simulink model "Mmc"  (R2024b)
settings: Solver=ode23t  StartTime=0.0  StopTime=2  FixedStep=Ts_Power
values from neighbouring files (symbols this model uses):
  Ch = 0.94e-6*ones(4,3)    [MmcParameters.m]
  Cm = 0.55e-3    (= 0.00055)    [MmcParameters.m]
  Cmo = 0.55e-3*ones(4,3)    [MmcParameters.m]
  eta = N*delta_wmax*Vmax^2/(P_rated*sin(phi_r)-Q_rated*cos(phi_r))    [MmcParameters.m]
  Fnom = 50    [MmcParameters.m]
  fs = 20000    [MmcParameters.m]
  I_b = Snom/Vnom_AC/sqrt(3)    [MmcParameters.m]
  Ipp_b = Snom/Vnom_AC/sqrt(3/2)    [MmcParameters.m]
  kicir = R0*alpha_ic    (= 62831.8530718)    [MmcParameters.m]
  kpcir = L0*alpha_ic    (= 1012.64003201)    [MmcParameters.m]
  L0 = (4.67e-3+5e-3)    (= 0.00967)    [MmcParameters.m]
  mu = eta*4/((2*Vmax^2-V0^2)^2-V0^4)*(P_rated*cos(phi_r)+Q_rated*sin(phi_r))/N    [MmcParameters.m]
  Nb_PM = 2    [MmcParameters.m]
  phi_r = pi/2    (= 1.57079632679)    [MmcParameters.m]
  R0 = 0.1+0.5    (= 0.6)    [MmcParameters.m]
  Rdis = 1e6*ones(4,3)    [MmcParameters.m]
  Rh = 1e-3./(2*pi*1000*Ch)    [MmcParameters.m]
  Rm = 0.2./(2*pi*120*Cmo)    [MmcParameters.m]
  SCR = 10    [MmcParameters.m]
  SigmaM = 10    [MmcParameters.m]
  Snom = 20*Vnom_AC*sqrt(3)    [MmcParameters.m]
  Ts_Power = 5e-7    (= 5e-07)    [MmcParameters.m]
  V0 = 1    [MmcParameters.m]
  V_b = Vnom_AC    (= 400)    [MmcParameters.m]
  VDCm = 480/2    (= 240)    [MmcParameters.m]
  VDCp = 480/2    (= 240)    [MmcParameters.m]
  Vnom_AC = 400    [MmcParameters.m]
  Vnom_PM = 480/2    (= 240)    [MmcParameters.m]
  w_b = 2*pi*Fnom    (= 314.159265359)    [MmcParameters.m]
  Zn = Vnom_AC^2 / Snom    [MmcParameters.m]
undefined symbols (not defined in the file or in its folder): DiscIntNeverNeededParam
libraries: spsIGBTDiodeLib x48, spsSeriesRLCBranchLib x42, spsVoltageMeasurementLib x16, spsTriangleGeneratorLib x12, spsCurrentMeasurementLib x7, spsFirstOrderFilterLib x6, eePwmGeneratorMultilevel x6, spsabctodq0Lib x3, spsGroundLib x2, spsMeanLib x2, spsDCVoltageSourceLib x2, spsThreePhaseVIMeasurementLib x2
(part 1 of 3)
settings Model: Creator=The MathWorks, Inc.  LastModifiedBy=isabe
settings SolverCC: AlgebraicLoopSolver=TrustRegion
settings DataIOCC: SaveFormat=StructureWithTime  SaveOutput=off  SignalLogging=off  DSMLogging=off  SaveTime=off  ReturnWorkspaceOutputs=off
settings OptimizationCC: ExpressionDepthLimit=2147483647  LifeSpan=inf
settings DebuggingCC: UnderspecifiedInitializationDetection=Classic  MergeDetectMultiDrivingBlocksExec=none  SolverPrmCheckMsg=warning  FcnCallInpInsideContextMsg=warning  UnconnectedInputMsg=warning  UnconnectedOutputMsg=warning  UnconnectedLineMsg=warning  AllowSymbolicDim=off  StateNameClashWarn=warning  SFUnexpectedBacktrackingDiag=warning  SFNoUnconditionalDefaultTransitionDiag=warning  SFExecutionAtInitializationDiag=none  ArithmeticOperatorsInVariantConditions=warning
settings HardwareCC: ProdBitPerPointer=32  ProdBitPerSizeT=32  ProdBitPerPtrDiffT=32  ProdLargestAtomicFloat=None  ProdIntDivRoundTo=Undefined  ProdEndianess=Unspecified  ProdWordSize=32  ProdHWDeviceType=32-bit Generic
settings ModelReferenceCC: EnableRefExpFcnMdlSchedulingChecks=on  PropagateSignalLabelsOutOfModel=off
settings SFSimCC: SimUseLocalCustomCode=off  CustomCodeUndefinedFunction=UseInterfaceOnly
settings RTWCC: RTWUseLocalCustomCode=off  GPUComputeCapability=3.5
settings CodeAppCC: StateflowObjectComments=on
settings GRTTargetCC: TargetLangStandard=C89/C90 (ANSI)  CombineOutputUpdateFcns=off  GRTInterface=on
settings ConfigComp: CovMetricSettings=dw  CovSaveCumulativeToWorkspaceVar=on  CovSaveSingleToWorkspaceVar=on  CovExternalEMLEnable=off
settings SimscapeCC: SimscapeNormalizeSystem=off  SimscapeNominalValues={1, 'bar'; 1, 'cm^3/s'; 1, 'bar*kg/s'; 1, 'kJ/kg'; 1, 'kW'; }

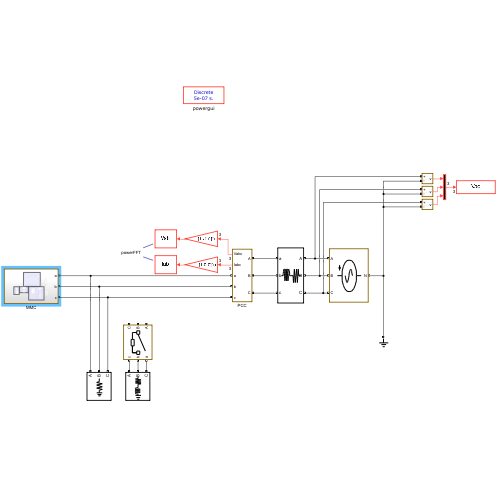
[thumbnail: Simulink's stored preview of the top-level diagram]
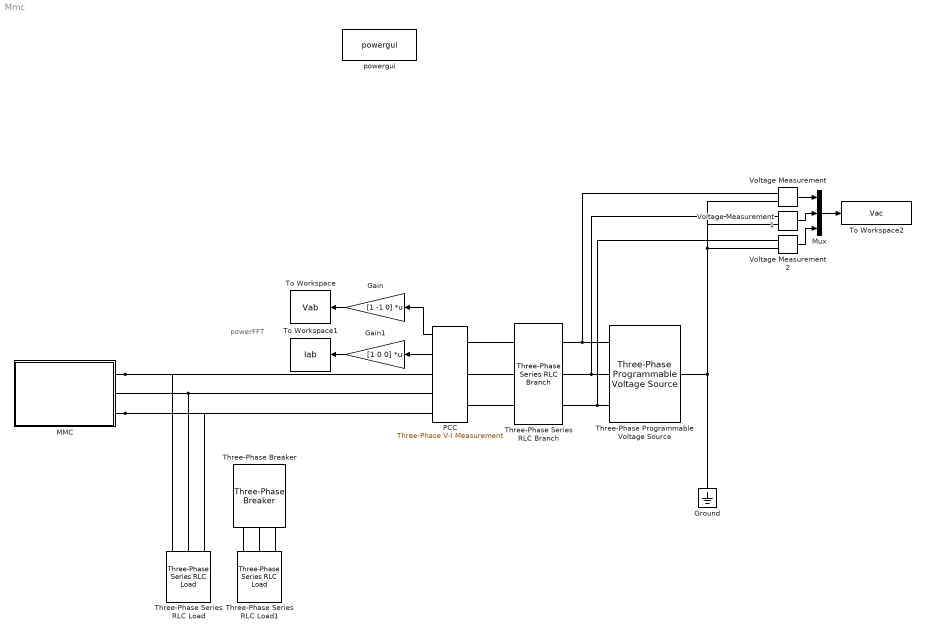
== system Mmc ==
  note: powerFFT
  Gain : Gain  Gain=[1 -1 0]  Multiplication=Matrix(K*u)
  Gain1 : Gain  Gain=[1 0 0]  Multiplication=Matrix(K*u)
  Ground : spsGroundLib/Ground  LConnTagsString=a
  MMC : Subsystem
  Mux : Mux  Inputs=3
  PCC : spsThreePhaseVIMeasurementLib/Three-Phase V-I Measurement  VoltageMeasurement=phase-to-ground  SetLabelV=off  LabelV=Vabc  Vpu=on  VpuLL=off  CurrentMeasurement=yes  SetLabelI=off  LabelI=Iabc  Ipu=on  Pbase=Snom  Vbase=Vnom_AC  OutputType=Complex  PhasorSimulation=off  PSBequivalent=0
  Three-Phase Programmable Voltage Source : spsThreePhaseProgrammableVoltageSourceLib/Three-Phase Programmable Voltage Source  PositiveSequence="[Vnom_AC  0 Fnom]"  VariationEntity=None  VariationType=Step  VariationTypeAlt=Step  VariationStep=-0.7  VariationRate=5  VariationMagnitude=0.3  VariationFrequency=2  VariationTiming=[1 17]  VariationPhaseA=off  Amplitudes=[1 0.8 1.2 1.0]  TimeValues=[0 0.1 0.15 0.2]  HarmonicGeneration=off  HarmonicA=[3 0.2 -25 0]  HarmonicB=[2 0.15 35 2]  Timing="[0.05  3]"  BusType=swing  Pref=0  Qref=0  Qmin=-inf  Qmax=inf
  Three-Phase Series RLC Branch : spsThreePhaseSeriesRLCBranchLib/Three-Phase Series RLC Branch  LConnTagsString=A|B|C  RConnTagsString=A|B|C  BranchType=RL  Resistance=Zn/SCR/sqrt(101)  Inductance=Zn/SCR/2/pi/Fnom*10/sqrt(101)  Capacitance=1e-6  Measurements=None
  Three-Phase Series RLC Load : spsThreePhaseSeriesRLCLoadLib/Three-Phase Series RLC Load  LConnTagsString=A|B|C  Configuration=Y (grounded)  NominalVoltage=Vnom_AC  Vabc=[1e3 1e3 1e3]  Vabcp=[1e3 1e3 1e3]  NominalFrequency=Fnom  UnbalancedPower=off  ActivePower=Snom*.05  InductivePower=Snom*.0  CapacitivePower=0  Pabc=[10e3 9e3 11e3]  QLabc=[100 90 110]  QCabc=[100 90 110]  Pabcp=[10e3 9e3 11e3]  QLabcp=[100 90 110]  QCabcp=[100 90 110]  Measurements=None  LoadType=constant Z
  Three-Phase Series RLC Load1 : spsThreePhaseSeriesRLCLoadLib/Three-Phase Series RLC Load  LConnTagsString=A|B|C  Configuration=Y (grounded)  NominalVoltage=Vnom_AC  Vabc=[1e3 1e3 1e3]  Vabcp=[1e3 1e3 1e3]  NominalFrequency=Fnom  UnbalancedPower=off  ActivePower=Snom*.25  InductivePower=Snom*.2  CapacitivePower=0  Pabc=[10e3 9e3 11e3]  QLabc=[100 90 110]  QCabc=[100 90 110]  Pabcp=[10e3 9e3 11e3]  QLabcp=[100 90 110]  QCabcp=[100 90 110]  Measurements=None  LoadType=constant PQ
  Three-Phase Breaker : spsThreePhaseBreakerLib/Three-Phase Breaker  InitialState=open  SwitchA=on  SwitchB=on  SwitchC=on  SwitchTimes=[.5 10]  External=off  BreakerResistance=1e-5  SnubberResistance=1e8  SnubberCapacitance=inf  Measurements=None
  To Workspace : ToWorkspace  VariableName=Vab  SaveFormat=Structure With Time  SampleTime=-1
      settings: Save2DSignal=2-D array (concatenate along first dimension)
  To Workspace1 : ToWorkspace  VariableName=Iab  SaveFormat=Structure With Time  SampleTime=-1
      settings: Save2DSignal=2-D array (concatenate along first dimension)
  To Workspace2 : ToWorkspace  VariableName=Vac  SaveFormat=Structure With Time  SampleTime=-1
  Voltage Measurement : spsVoltageMeasurementLib/Voltage Measurement  PhasorSimulation=off  OutputType=Complex  PSBequivalent=0
  Voltage Measurement1 : spsVoltageMeasurementLib/Voltage Measurement  PhasorSimulation=off  OutputType=Complex  PSBequivalent=0
  Voltage Measurement2 : spsVoltageMeasurementLib/Voltage Measurement  PhasorSimulation=off  OutputType=Complex  PSBequivalent=0
  powergui : sps_lib/powergui  Priority=1  SimulationMode=Discrete  SampleTime=Ts_Power  frequency=60  Iterations=50  frequencyindice=0  Pbase=100e6  ErrMax=1e-4  UnitsV=kV  UnitsW=MW  buscounter=0  FunctionMessages=off  echomessages=off  EnableUseOfTLC=off  CurrentSourceSwitches=off  DisableSnubberDevices=off  DisableRonSwitches=off  DisableVfSwitches=off  DisplayEquations=off  AutomaticDiscreteSolvers=off  SolverType=Tustin/Backward Euler (TBE)  Interpol=off  ExternalGateDelay=off  methode=off  Ts=10  x0status=blocks  SPID=off  SwTol=0  HookPort=off  NonlinearTolerance=1e-4  nMaxIteration=100  ContinueOnMaxIteration=off  RestoreLinks=warning  ResistiveCurrentMeasurement=off  Frange=[0:2:500]  Ylog=off  Xlog=on  ShowGrid=off  save=off  variable=ZData  structure=Vout  ZoomFFT=on  StartTime=0.15  cycles=2  DisplayStyle=1  fundamental=50  FreqAxis=on  MaxFrequency=6000  frequencyindicesteady=1  RmsSteady=1  display=off
  wires:
  PCC/1 -> Gain/1
  Gain/1 -> To Workspace/1
  PCC/2 -> Gain1/1
  Gain1/1 -> To Workspace1/1
  Voltage Measurement/1 -> Mux/1
  Voltage Measurement1/1 -> Mux/2
  Voltage Measurement2/1 -> Mux/3
  Mux/1 -> To Workspace2/1
  connections:
  Three-Phase Series RLC Branch/LConn1 -- Voltage Measurement/LConn1 -- Three-Phase Programmable Voltage Source/RConn1
  Three-Phase Series RLC Branch/LConn2 -- Three-Phase Programmable Voltage Source/RConn2 -- Voltage Measurement1/LConn1
  Three-Phase Series RLC Branch/LConn3 -- Voltage Measurement2/LConn1 -- Three-Phase Programmable Voltage Source/RConn3
  Ground/LConn1 -- Voltage Measurement/LConn2 -- Voltage Measurement1/LConn2 -- Voltage Measurement2/LConn2 -- Three-Phase Programmable Voltage Source/LConn1
  MMC/LConn1 -- Three-Phase Series RLC Load/LConn1 -- PCC/RConn1
  Three-Phase Series RLC Load/LConn2 -- PCC/RConn2 -- MMC/LConn2
  MMC/LConn3 -- Three-Phase Series RLC Load/LConn3 -- PCC/RConn3
  Three-Phase Series RLC Load1/LConn1 -- Three-Phase Breaker/RConn3
  Three-Phase Series RLC Load1/LConn2 -- Three-Phase Breaker/RConn2
  Three-Phase Series RLC Load1/LConn3 -- Three-Phase Breaker/RConn1
  PCC/LConn1 -- Three-Phase Series RLC Branch/RConn1
  PCC/LConn2 -- Three-Phase Series RLC Branch/RConn2
  PCC/LConn3 -- Three-Phase Series RLC Branch/RConn3

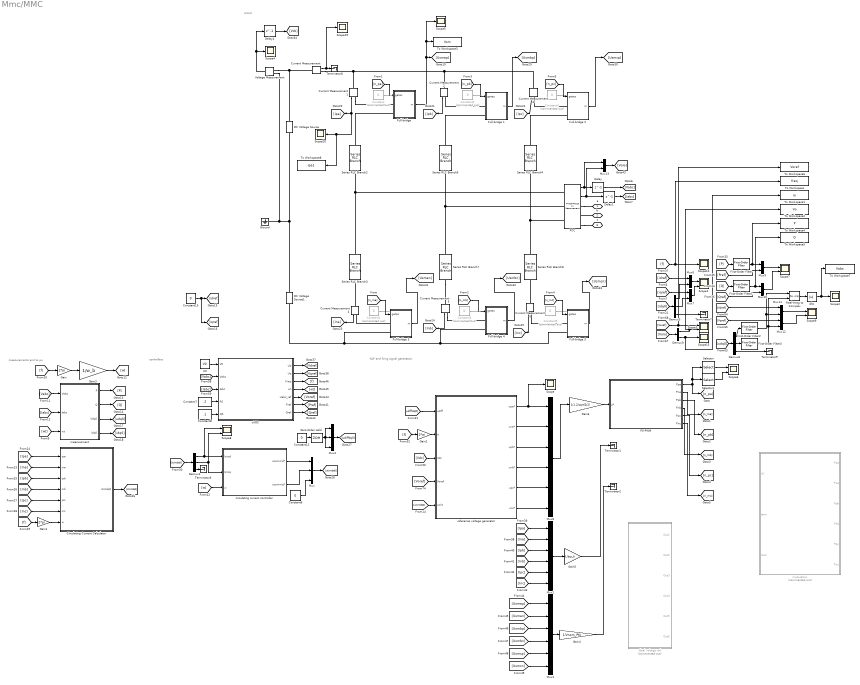
== system Mmc/MMC ==
  note: controllers
  note: circuit
  note: NLP and firing signal generation
  note: measurements and to pu
  Abs : Abs  SaturateOnIntegerOverflow=off
  Circulating Current Calculator : Subsystem
  Constant{,1..5} (6 alike) : Constant  Commented=on  Value=0
  Constant12 : Constant  Value=0
  Constant13 : Constant  Value=0
  Constant6 : Constant  Value=0
  Constant7 : Constant  Value=.2
  Constant8 : Constant  Value=.1
  Current Measurement{,1..6} (7 alike) : spsCurrentMeasurementLib/Current Measurement  PhasorSimulation=off  OutputType=Complex  PSBequivalent=0
  DC Voltage Source : spsDCVoltageSourceLib/DC Voltage Source  Amplitude=VDCp  Measurements=None
  DC Voltage Source1 : spsDCVoltageSourceLib/DC Voltage Source  Amplitude=VDCm  Measurements=None
  Delay : Delay  DelayLength=1  SampleTime=Ts_Power
  Delay1 : Delay  DelayLength=1  SampleTime=Ts_Power
  Delay4 : Delay  DelayLength=1  InputProcessing=Columns as channels (frame based)
  Demux2 : Demux  Outputs=3
  Demux3 : Demux  Outputs=3
  Demux8 : Demux  Outputs=3
  Demux9 : Demux  Outputs=2
  First-Order Filter : spsFirstOrderFilterLib/First-Order Filter  FilterType=Lowpass  Tc=1/120  Ts=Ts_Power  Initialize=on  Vac_Init=[0, 0, 60]  Vdc_Init=0  PlotResponse=off  FreqRange="[0,  200,  1]"
  First-Order Filter1 : spsFirstOrderFilterLib/First-Order Filter  FilterType=Lowpass  Tc=1/120  Ts=Ts_Power  Initialize=on  Vac_Init=[0, 0, 60]  Vdc_Init=0  PlotResponse=off  FreqRange="[0,  200,  1]"
  First-Order Filter2 : spsFirstOrderFilterLib/First-Order Filter  FilterType=Lowpass  Tc=1/120  Ts=Ts_Power  Initialize=on  Vac_Init=[0, 0, 60]  Vdc_Init=1  PlotResponse=off  FreqRange="[0,  200,  1]"
  First-Order Filter3 : spsFirstOrderFilterLib/First-Order Filter  FilterType=Lowpass  Tc=1/120  Ts=Ts_Power  Initialize=on  Vac_Init=[0, 0, 60]  Vdc_Init=0  PlotResponse=off  FreqRange="[0,  200,  1]"
  Full-bridge : Subsystem
  Full-bridge 1 : Subsystem
  Full-bridge 2 : Subsystem
  Full-bridge 3 : Subsystem
  Full-bridge 4 : Subsystem
  Full-bridge 5 : Subsystem
  Gain : Gain  Gain=2*pi
  Gain1 : Gain  Gain=2*pi
  Gain2 : Gain  Gain=2*pi
  Gain3 : Gain  Gain=1/w_b
  Gain4 : Gain  Gain=1/Vnom_PM
  Gain5 : Gain  Gain=1/Ipp_b
  Gain6 : Gain  Gain=1/1.2/sqrt(3/2)
  Ground : spsGroundLib/Ground  LConnTagsString=a
  Ideal voltage ref : Subsystem  Commented=on
  Mux : Mux  Inputs=3
  Mux{6..7,9..13} (7 alike) : Mux  Inputs=2
  Mux2 : Mux  Inputs=6
  Mux3 : Mux  Inputs=6
  Mux4 : Mux  Inputs=3
  Mux8 : Mux  Inputs=6
  PCC : spsThreePhaseVIMeasurementLib/Three-Phase V-I Measurement  VoltageMeasurement=phase-to-ground  SetLabelV=off  LabelV=Vabc  Vpu=on  VpuLL=off  CurrentMeasurement=yes  SetLabelI=off  LabelI=Iabc  Ipu=on  Pbase=Snom  Vbase=Vnom_AC  OutputType=Complex  PhasorSimulation=off  PSBequivalent=0
  PS-PWM : Subsystem
  Real-Imag to Complex : RealImagToComplex
  Scope{,2,4..5,10,15,19..20} (8 alike) : Scope
  Scope{1,3,6..9} (6 alike) : Scope  NumInputPorts=2
  Selector : Selector  InputPortWidth=2*Nb_PM  IndexOptions=Index vector (dialog)  Indices=[1]  OutputSizes=1
  Selector1 : Selector  InputPortWidth=2*Nb_PM  IndexOptions=Index vector (dialog)  Indices=[Nb_PM]  OutputSizes=1
  Series RLC Branch{2..4,6..8} (6 alike) : spsSeriesRLCBranchLib/Series RLC Branch  LConnTagsString=__new0  RConnTagsString=__new0  BranchType=RL  Resistance=R0  Inductance=L0  SetiL0=off  InitialCurrent=0  Capacitance=1e-6  Setx0=off  InitialVoltage=0  Measurements=None
  Terminator{1..2,6..9} (6 alike) : Terminator
  To Workspace : ToWorkspace  VariableName=freq  SaveFormat=Structure With Time  SampleTime=-1
  To Workspace1 : ToWorkspace  VariableName=Io  SaveFormat=Structure With Time  SampleTime=-1
  To Workspace2 : ToWorkspace  VariableName=Vo  SaveFormat=Structure With Time  SampleTime=-1
  To Workspace3 : ToWorkspace  VariableName=Vsm  SaveFormat=Structure With Time  SampleTime=-1
  To Workspace4 : ToWorkspace  VariableName=P  SaveFormat=Structure With Time  SampleTime=-1
  To Workspace5 : ToWorkspace  VariableName=Q  SaveFormat=Structure With Time  SampleTime=-1
  To Workspace6 : ToWorkspace  VariableName=Voref  SaveFormat=Structure With Time  SampleTime=-1
  To Workspace7 : ToWorkspace  VariableName=Vabs  SaveFormat=Structure With Time  SampleTime=-1
  To Workspace8 : ToWorkspace  VariableName=Ipa1  SaveFormat=Structure With Time  SampleTime=-1
  U0 : Constant  Value=V0  SampleTime=Ts_Power
  Voltage Measurement : spsVoltageMeasurementLib/Voltage Measurement  PhasorSimulation=off  OutputType=Complex  PSBequivalent=0
  Zero-Order Hold : ZeroOrderHold  SampleTime=Ts_Power
  circulating current controller : Subsystem
  measurement : Subsystem
  modulation : Subsystem  Commented=on
  reference voltage generator : Subsystem
  uVOC : Subsystem
  a : PMIOPort  Side=Left
  b : PMIOPort  Port=2  Side=Left
  c : PMIOPort  Port=3  Side=Left
  wires:
  Constant4/1 -> ?
  [n_pc] -> Full-bridge 2/1(gates)
  [n_pb] -> Full-bridge 1/1(gates)
  [n_pa] -> Full-bridge/1(gates)
  [n_mb] -> Full-bridge 4/1(gates)
  Constant1/1 -> ?
  Constant3/1 -> ?
  Full-bridge/1(m) -> To Workspace3/1, Scope5/1, [Usmap]
  Constant2/1 -> ?
  Constant/1 -> ?
  [n_ma] -> Full-bridge 3/1(gates)
  Constant5/1 -> ?
  [n_mc] -> Full-bridge 5/1(gates)
  PCC/1 -> Mux13/1, Delay/1
  PCC/2 -> Mux13/2, Delay1/1
  [Vabc] -> measurement/1(Vabc)
  [Iabc] -> measurement/2(Iabc)
  [wt] -> measurement/3(wt)
  [f] -> Gain/1
  Gain/1 -> Gain3/1
  Gain3/1 -> [w]
  circulating current controller/1(ucommd*) -> Mux/1
  circulating current controller/2(ucommq*) -> Mux/2
  Constant6/1 -> Mux/3
  measurement/1(P) -> [P]
  measurement/3(Vdq0) -> [udq0]
  measurement/4(Idq0) -> [idq0]
  [w] -> circulating current controller/3(w)
  Current Measurement1/1 -> To Workspace8/1, Scope20/1, [Ipa]
  Current Measurement2/1 -> [Ipb]
  Current Measurement3/1 -> [Ipc]
  Current Measurement4/1 -> [Ina]
  Current Measurement5/1 -> [Inb]
  Current Measurement6/1 -> [Inc]
  [Ipa] -> Circulating Current Calculator/1(ipa)
  [Ina] -> Circulating Current Calculator/2(ina)
  [Ipb] -> Circulating Current Calculator/3(ipb)
  [Inb] -> Circulating Current Calculator/4(inb)
  [Ipc] -> Circulating Current Calculator/5(ipc)
  [Inc] -> Circulating Current Calculator/6(inc)
  [f] -> Gain1/1
  Gain1/1 -> Circulating Current Calculator/7(w)
  Circulating Current Calculator/1(icircdq0) -> [Icircdq0]
  [Icircdq0] -> Demux2/1
  Demux2/1 -> Scope8/1, circulating current controller/1(Icircd)
  Demux2/2 -> circulating current controller/2(Icircq), Scope8/2
  Demux2/3 -> Terminator6/1
  [f] -> Gain2/1
  measurement/2(Q) -> [Q]
  Delay/1 -> [Vabc]
  Delay1/1 -> [Iabc]
  PS-PWM/1(Ppa) -> [n_pa], Selector1/1, Selector/1
  PS-PWM/2(Pna) -> [n_ma]
  PS-PWM/3(Ppb) -> [n_pb]
  PS-PWM/4(Pnb) -> [n_mb]
  PS-PWM/5(Ppc) -> [n_pc]
  PS-PWM/6(Pnc) -> [n_mc]
  [idq0] -> Demux3/1
  Demux3/3 -> Terminator7/1
  [idref] -> Mux6/1
  Demux3/1 -> Mux6/2
  [iqref] -> Mux7/1
  Demux3/2 -> Mux7/2
  Mux/1 -> [ucircdq0]
  [P] -> First-Order Filter/1
  [Pref] -> Mux9/2
  [Q] -> First-Order Filter1/1
  [Qref] -> Mux10/2
  reference voltage generator/1(upa*) -> Scope/1, Mux8/1
  reference voltage generator/2(una*) -> Mux8/2
  reference voltage generator/3(upb*) -> Mux8/3
  reference voltage generator/4(unb*) -> Mux8/4
  reference voltage generator/5(upc*) -> Mux8/5
  reference voltage generator/6(unc*) -> Mux8/6
  [Ipa] -> Mux2/1
  [Ina] -> Mux2/2
  [Ipb] -> Mux2/3
  [Inb] -> Mux2/4
  [Ipc] -> Mux2/5
  [Inc] -> Mux2/6
  Mux2/1 -> Gain5/1
  Current Measurement/1 -> Scope19/1, Terminator8/1
  Full-bridge 1/1(m) -> [Usmbp]
  Full-bridge 2/1(m) -> [Usmcp]
  Full-bridge 3/1(m) -> [Usman]
  Full-bridge 4/1(m) -> [Usmbn]
  Full-bridge 5/1(m) -> [Usmcn]
  [Usmap] -> Mux3/1
  [Usman] -> Mux3/2
  [Usmbp] -> Mux3/3
  [Usmbn] -> Mux3/4
  [Usmcp] -> Mux3/5
  Mux3/1 -> Gain4/1
  [Usmcn] -> Mux3/6
  Gain4/1 -> Terminator2/1
  Gain5/1 -> Terminator1/1
  Selector/1 -> Scope6/1
  Selector1/1 -> Scope6/2
  Voltage Measurement/1 -> Delay4/1, Scope4/1
  Delay4/1 -> [Vdc]
  Mux6/1 -> Scope1/1
  Mux7/1 -> Scope1/2
  [udq0] -> Demux8/1
  Demux8/3 -> Terminator9/1
  [Vdref] -> Mux11/1
  Demux8/1 -> First-Order Filter2/1
  [Vqref] -> Mux12/1
  Demux8/2 -> First-Order Filter3/1
  Mux13/1 -> [VoIo]
  [VoIo] -> Demux9/1
  Demux9/1 -> To Workspace2/1, Scope3/2
  [f] -> To Workspace/1, Scope10/1
  [Voref] -> reference voltage generator/4(Voref)
  [ucircdq0] -> reference voltage generator/5(ucirc)
  [udiffdq0] -> reference voltage generator/1(udiff)
  [Vdc] -> reference voltage generator/3(Vdc)
  Demux9/2 -> To Workspace1/1, Scope15/1
  Mux8/1 -> Gain6/1
  U0/1 -> uVOC/1(V0)
  [Vabc] -> uVOC/2(Vabc)
  [Iabc] -> uVOC/3(Iabc)
  Constant7/1 -> uVOC/4(P0)
  Constant8/1 -> uVOC/5(Q0)
  uVOC/1(Ud) -> [Vdref]
  uVOC/6(Pref) -> [Pref]
  uVOC/2(Uq) -> [Vqref]
  uVOC/3(Freq) -> [f]
  uVOC/4(wt) -> [wt]
  uVOC/7(Qref) -> [Qref]
  uVOC/5(Uabc_ref) -> [Voref]
  Gain6/1 -> PS-PWM/1(U*)
  Constant12/1 -> Zero-Order Hold/1
  Zero-Order Hold/1 -> Mux4/3, Mux4/1, Mux4/2
  Mux4/1 -> [udiffdq0]
  Constant13/1 -> [idref], [iqref]
  Mux9/1 -> Scope7/1
  Mux10/1 -> Scope7/2
  [Voref] -> Scope3/1, To Workspace6/1
  Mux11/1 -> Scope9/1
  Mux12/1 -> Scope9/2
  First-Order Filter/1 -> To Workspace4/1, Mux9/1
  First-Order Filter1/1 -> To Workspace5/1, Mux10/1
  First-Order Filter2/1 -> Real-Imag to Complex/1, Mux11/2
  First-Order Filter3/1 -> Real-Imag to Complex/2, Mux12/2
  Real-Imag to Complex/1 -> Abs/1
  Abs/1 -> To Workspace7/1, Scope2/1
  Gain2/1 -> reference voltage generator/2(w)
  connections:
  DC Voltage Source1/LConn1 -- Full-bridge 5/LConn2 -- Full-bridge 4/LConn2 -- Full-bridge 3/LConn2
  Full-bridge 2/LConn2 -- Series RLC Branch4/LConn1
  Current Measurement/RConn1 -- Current Measurement2/LConn1 -- Current Measurement3/LConn1 -- Current Measurement1/LConn1
  Series RLC Branch8/LConn1 -- PCC/LConn3 -- Series RLC Branch4/RConn1
  Series RLC Branch2/LConn1 -- Full-bridge/LConn2
  Series RLC Branch3/LConn1 -- Series RLC Branch2/RConn1 -- PCC/LConn1
  Full-bridge 1/LConn2 -- Series RLC Branch6/LConn1
  Series RLC Branch7/LConn1 -- Series RLC Branch6/RConn1 -- PCC/LConn2
  PCC/RConn1 -- a/RConn1
  b/RConn1 -- PCC/RConn2
  PCC/RConn3 -- c/RConn1
  Current Measurement/LConn1 -- DC Voltage Source/RConn1 -- Voltage Measurement/LConn1
  Current Measurement1/RConn1 -- Full-bridge/LConn1
  Full-bridge 1/LConn1 -- Current Measurement2/RConn1
  Full-bridge 2/LConn1 -- Current Measurement3/RConn1
  Full-bridge 3/LConn1 -- Current Measurement4/RConn1
  Current Measurement4/LConn1 -- Series RLC Branch3/RConn1
  Series RLC Branch7/RConn1 -- Current Measurement5/LConn1
  Current Measurement5/RConn1 -- Full-bridge 4/LConn1
  Current Measurement6/LConn1 -- Series RLC Branch8/RConn1
  Current Measurement6/RConn1 -- Full-bridge 5/LConn1
  Voltage Measurement/LConn2 -- Ground/LConn1 -- DC Voltage Source1/RConn1 -- DC Voltage Source/LConn1

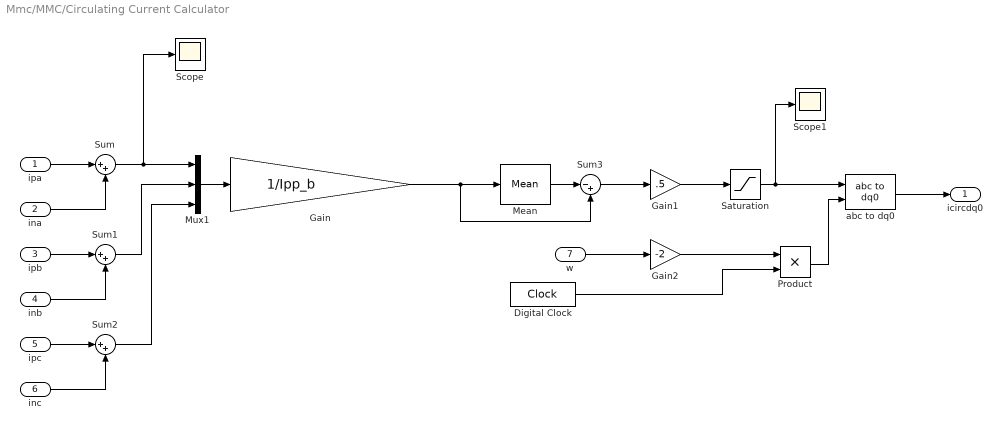
== system Mmc/MMC/Circulating Current Calculator ==
  ipa : Inport
  ina : Inport  Port=2
  ipb : Inport  Port=3
  inb : Inport  Port=4
  ipc : Inport  Port=5
  inc : Inport  Port=6
  w : Inport  Port=7
  Digital Clock : DigitalClock  SampleTime=Ts_Power
  Gain : Gain  Gain=1/Ipp_b
  Gain1 : Gain  Gain=.5
  Gain2 : Gain  Gain=-2
  Mean : spsMeanLib/Mean  Freq=Fnom*2*2  Vinit=0  Ts=Ts_Power
  Mux1 : Mux  Inputs=3
  Product : Product
  Saturation : Saturate  UpperLimit=1.2  LowerLimit=-1.2
  Scope : Scope
  Scope1 : Scope
  Sum : Sum  Inputs=|++
  Sum1 : Sum  Inputs=|++
  Sum2 : Sum  Inputs=|++
  Sum3 : Sum  Inputs=|-+
  abc to dq0 : spsabctodq0Lib/abc to dq0  Alignment=90 degrees behind phase A axis
  icircdq0 : Outport
  wires:
  Sum2/1 -> Mux1/3
  ina/1 -> Sum/2
  Mux1/1 -> Gain/1
  ipb/1 -> Sum1/1
  Sum/1 -> Scope/1, Mux1/1
  Sum1/1 -> Mux1/2
  ipc/1 -> Sum2/1
  inb/1 -> Sum1/2
  ipa/1 -> Sum/1
  inc/1 -> Sum2/2
  Gain1/1 -> Saturation/1
  abc to dq0/1 -> icircdq0/1
  w/1 -> Gain2/1
  Gain2/1 -> Product/1
  Digital Clock/1 -> Product/2
  Product/1 -> abc to dq0/2
  Mean/1 -> Sum3/1
  Sum3/1 -> Gain1/1
  Gain/1 -> Mean/1, Sum3/2
  Saturation/1 -> Scope1/1, abc to dq0/1

== system Mmc/MMC/Full-bridge ==
  gates : Inport
  Demux : Demux
  HBua1 : Subsystem
  HBua2 : Subsystem
  Mux : Mux
  Mux1 : Mux
  Mux2 : Mux  Inputs=2
  vm : spsVoltageMeasurementLib/Voltage Measurement  PhasorSimulation=off  OutputType=Complex  PSBequivalent=0
  vm1 : spsVoltageMeasurementLib/Voltage Measurement  PhasorSimulation=off  OutputType=Complex  PSBequivalent=0
  VA : PMIOPort  Side=Left
  VB : PMIOPort  Port=2  Side=Left
  m : Outport
  wires:
  Mux1/1 -> HBua2/1(gates)
  gates/1 -> Demux/1
  Mux/1 -> HBua1/1(gates)
  vm/1 -> Mux2/1
  vm1/1 -> Mux2/2
  Mux2/1 -> m/1
  Demux/1 -> Mux/4, Mux/1
  Demux/2 -> Mux/3, Mux/2
  Demux/3 -> Mux1/4, Mux1/1
  Demux/4 -> Mux1/3, Mux1/2
  connections:
  HBua1/LConn1 -- VA/RConn1
  HBua2/LConn2 -- VB/RConn1
  vm/LConn1 -- HBua1/RConn1
  HBua1/LConn2 -- HBua2/LConn1
  HBua2/RConn1 -- vm1/LConn1
  vm/LConn2 -- HBua1/RConn2
  HBua2/RConn2 -- vm1/LConn2

== system Mmc/MMC/Full-bridge 1 ==
  gates : Inport
  Demux : Demux
  HBua1 : Subsystem
  HBua2 : Subsystem
  Mux : Mux
  Mux1 : Mux
  Mux2 : Mux  Inputs=2
  vm : spsVoltageMeasurementLib/Voltage Measurement  PhasorSimulation=off  OutputType=Complex  PSBequivalent=0
  vm1 : spsVoltageMeasurementLib/Voltage Measurement  PhasorSimulation=off  OutputType=Complex  PSBequivalent=0
  VA : PMIOPort  Side=Left
  VB : PMIOPort  Port=2  Side=Left
  m : Outport
  wires:
  Mux1/1 -> HBua2/1(gates)
  gates/1 -> Demux/1
  Mux/1 -> HBua1/1(gates)
  vm/1 -> Mux2/1
  vm1/1 -> Mux2/2
  Mux2/1 -> m/1
  Demux/1 -> Mux/4, Mux/1
  Demux/2 -> Mux/3, Mux/2
  Demux/3 -> Mux1/4, Mux1/1
  Demux/4 -> Mux1/3, Mux1/2
  connections:
  HBua1/LConn1 -- VA/RConn1
  HBua2/LConn2 -- VB/RConn1
  vm/LConn1 -- HBua1/RConn1
  HBua1/LConn2 -- HBua2/LConn1
  HBua2/RConn1 -- vm1/LConn1
  vm/LConn2 -- HBua1/RConn2
  HBua2/RConn2 -- vm1/LConn2

== system Mmc/MMC/Full-bridge 2 ==
  gates : Inport
  Demux : Demux
  HBua1 : Subsystem
  HBua2 : Subsystem
  Mux : Mux
  Mux1 : Mux
  Mux2 : Mux  Inputs=2
  vm : spsVoltageMeasurementLib/Voltage Measurement  PhasorSimulation=off  OutputType=Complex  PSBequivalent=0
  vm1 : spsVoltageMeasurementLib/Voltage Measurement  PhasorSimulation=off  OutputType=Complex  PSBequivalent=0
  VA : PMIOPort  Side=Left
  VB : PMIOPort  Port=2  Side=Left
  m : Outport
  wires:
  Mux1/1 -> HBua2/1(gates)
  gates/1 -> Demux/1
  Mux/1 -> HBua1/1(gates)
  vm/1 -> Mux2/1
  vm1/1 -> Mux2/2
  Mux2/1 -> m/1
  Demux/1 -> Mux/4, Mux/1
  Demux/2 -> Mux/3, Mux/2
  Demux/3 -> Mux1/4, Mux1/1
  Demux/4 -> Mux1/3, Mux1/2
  connections:
  HBua1/LConn1 -- VA/RConn1
  HBua2/LConn2 -- VB/RConn1
  vm/LConn1 -- HBua1/RConn1
  HBua1/LConn2 -- HBua2/LConn1
  HBua2/RConn1 -- vm1/LConn1
  vm/LConn2 -- HBua1/RConn2
  HBua2/RConn2 -- vm1/LConn2

== system Mmc/MMC/Full-bridge 3 ==
  gates : Inport
  Demux : Demux
  HBua1 : Subsystem
  HBua2 : Subsystem
  Mux : Mux
  Mux1 : Mux
  Mux2 : Mux  Inputs=2
  vm : spsVoltageMeasurementLib/Voltage Measurement  PhasorSimulation=off  OutputType=Complex  PSBequivalent=0
  vm1 : spsVoltageMeasurementLib/Voltage Measurement  PhasorSimulation=off  OutputType=Complex  PSBequivalent=0
  VA : PMIOPort  Side=Left
  VB : PMIOPort  Port=2  Side=Left
  m : Outport
  wires:
  Mux1/1 -> HBua2/1(gates)
  gates/1 -> Demux/1
  Mux/1 -> HBua1/1(gates)
  vm/1 -> Mux2/1
  vm1/1 -> Mux2/2
  Mux2/1 -> m/1
  Demux/1 -> Mux/4, Mux/1
  Demux/2 -> Mux/3, Mux/2
  Demux/3 -> Mux1/4, Mux1/1
  Demux/4 -> Mux1/3, Mux1/2
  connections:
  HBua1/LConn1 -- VA/RConn1
  HBua2/LConn2 -- VB/RConn1
  vm/LConn1 -- HBua1/RConn1
  HBua1/LConn2 -- HBua2/LConn1
  HBua2/RConn1 -- vm1/LConn1
  vm/LConn2 -- HBua1/RConn2
  HBua2/RConn2 -- vm1/LConn2

== system Mmc/MMC/Full-bridge 4 ==
  gates : Inport
  Demux : Demux
  HBua1 : Subsystem
  HBua2 : Subsystem
  Mux : Mux
  Mux1 : Mux
  Mux2 : Mux  Inputs=2
  vm : spsVoltageMeasurementLib/Voltage Measurement  PhasorSimulation=off  OutputType=Complex  PSBequivalent=0
  vm1 : spsVoltageMeasurementLib/Voltage Measurement  PhasorSimulation=off  OutputType=Complex  PSBequivalent=0
  VA : PMIOPort  Side=Left
  VB : PMIOPort  Port=2  Side=Left
  m : Outport
  wires:
  Mux1/1 -> HBua2/1(gates)
  gates/1 -> Demux/1
  Mux/1 -> HBua1/1(gates)
  vm/1 -> Mux2/1
  vm1/1 -> Mux2/2
  Mux2/1 -> m/1
  Demux/1 -> Mux/4, Mux/1
  Demux/2 -> Mux/3, Mux/2
  Demux/3 -> Mux1/4, Mux1/1
  Demux/4 -> Mux1/3, Mux1/2
  connections:
  HBua1/LConn1 -- VA/RConn1
  HBua2/LConn2 -- VB/RConn1
  vm/LConn1 -- HBua1/RConn1
  HBua1/LConn2 -- HBua2/LConn1
  HBua2/RConn1 -- vm1/LConn1
  vm/LConn2 -- HBua1/RConn2
  HBua2/RConn2 -- vm1/LConn2

== system Mmc/MMC/Full-bridge 5 ==
  gates : Inport
  Demux : Demux
  HBua1 : Subsystem
  HBua2 : Subsystem
  Mux : Mux
  Mux1 : Mux
  Mux2 : Mux  Inputs=2
  vm : spsVoltageMeasurementLib/Voltage Measurement  PhasorSimulation=off  OutputType=Complex  PSBequivalent=0
  vm1 : spsVoltageMeasurementLib/Voltage Measurement  PhasorSimulation=off  OutputType=Complex  PSBequivalent=0
  VA : PMIOPort  Side=Left
  VB : PMIOPort  Port=2  Side=Left
  m : Outport
  wires:
  Mux1/1 -> HBua2/1(gates)
  gates/1 -> Demux/1
  Mux/1 -> HBua1/1(gates)
  vm/1 -> Mux2/1
  vm1/1 -> Mux2/2
  Mux2/1 -> m/1
  Demux/1 -> Mux/4, Mux/1
  Demux/2 -> Mux/3, Mux/2
  Demux/3 -> Mux1/4, Mux1/1
  Demux/4 -> Mux1/3, Mux1/2
  connections:
  HBua1/LConn1 -- VA/RConn1
  HBua2/LConn2 -- VB/RConn1
  vm/LConn1 -- HBua1/RConn1
  HBua1/LConn2 -- HBua2/LConn1
  HBua2/RConn1 -- vm1/LConn1
  vm/LConn2 -- HBua1/RConn2
  HBua2/RConn2 -- vm1/LConn2

== system Mmc/MMC/Ideal voltage ref ==
  Gain4 : Gain  Gain=-1
  Gain5 : Gain  Gain=-1
  Gain6 : Gain  Gain=-1
  Sine Wave : Sin  Amplitude=sqrt(3/2)  Frequency=50*2*pi  SampleTime=Ts_Power
  Sine Wave1 : Sin  Amplitude=Vnom_AC*sqrt(2/3)/Vnom_PM/Nb_PM  Frequency=50*2*pi  Phase=4*pi/3  SampleTime=Ts_Power
  Sine Wave2 : Sin  Amplitude=Vnom_AC*sqrt(2/3)/Vnom_PM/Nb_PM  Frequency=50*2*pi  Phase=2*pi/3  SampleTime=Ts_Power
  Out1 : Outport
  Out2 : Outport  Port=2
  Out3 : Outport  Port=3
  Out4 : Outport  Port=4
  Out5 : Outport  Port=5
  Out6 : Outport  Port=6
  wires:
  Gain4/1 -> Out2/1
  Sine Wave1/1 -> Out3/1, Gain5/1
  Sine Wave2/1 -> Out5/1, Gain6/1
  Sine Wave/1 -> Out1/1, Gain4/1
  Gain6/1 -> Out6/1
  Gain5/1 -> Out4/1

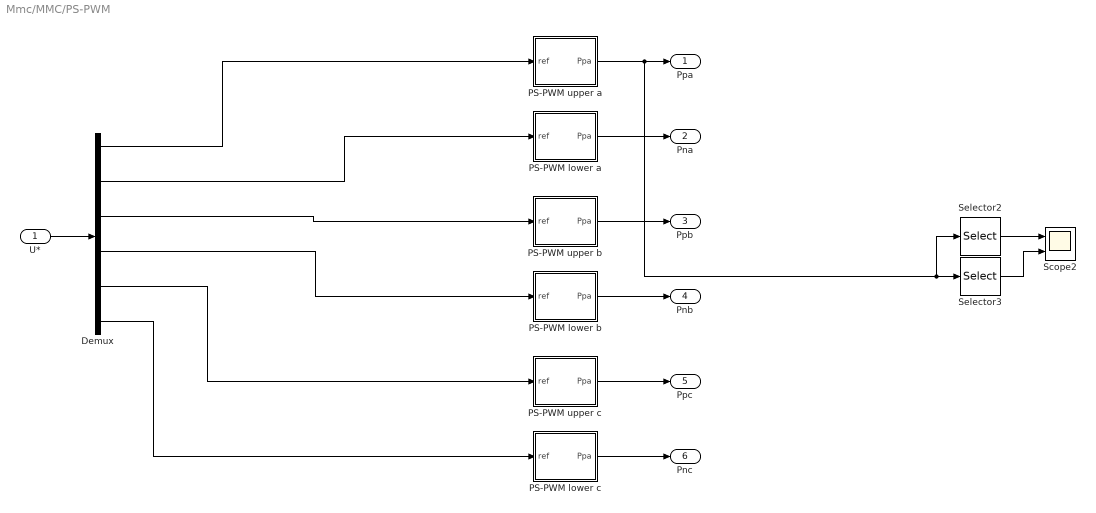
== system Mmc/MMC/PS-PWM ==
  U* : Inport
  Demux : Demux  Outputs=6
  PS-PWM lower a : Subsystem
  PS-PWM lower b : Subsystem
  PS-PWM lower c : Subsystem
  PS-PWM upper a : Subsystem
  PS-PWM upper b : Subsystem
  PS-PWM upper c : Subsystem
  Scope2 : Scope  NumInputPorts=2
  Selector2 : Selector  InputPortWidth=2*Nb_PM  IndexOptions=Index vector (dialog)  Indices=[1]  OutputSizes=1
  Selector3 : Selector  InputPortWidth=2*Nb_PM  IndexOptions=Index vector (dialog)  Indices=[Nb_PM]  OutputSizes=1
  Ppa : Outport
  Pna : Outport  Port=2
  Ppb : Outport  Port=3
  Pnb : Outport  Port=4
  Ppc : Outport  Port=5
  Pnc : Outport  Port=6
  wires:
  U*/1 -> Demux/1
  Demux/3 -> PS-PWM upper b/1(ref)
  Demux/4 -> PS-PWM lower b/1(ref)
  Demux/5 -> PS-PWM upper c/1(ref)
  Demux/6 -> PS-PWM lower c/1(ref)
  PS-PWM lower a/1(Ppa) -> Pna/1
  Demux/2 -> PS-PWM lower a/1(ref)
  PS-PWM upper c/1(Ppa) -> Ppc/1
  PS-PWM lower c/1(Ppa) -> Pnc/1
  PS-PWM lower b/1(Ppa) -> Pnb/1
  PS-PWM upper b/1(Ppa) -> Ppb/1
  Demux/1 -> PS-PWM upper a/1(ref)
  Selector2/1 -> Scope2/1
  Selector3/1 -> Scope2/2
  PS-PWM upper a/1(Ppa) -> Selector3/1, Selector2/1, Ppa/1

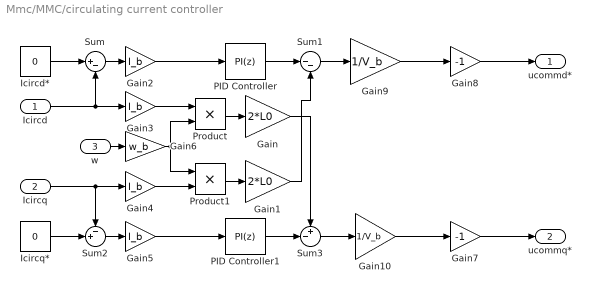
== system Mmc/MMC/circulating current controller ==
  Icircd : Inport
  Icircq : Inport  Port=2
  w : Inport  Port=3
  Gain : Gain  Gain=2*L0
  Gain1 : Gain  Gain=2*L0
  Gain10 : Gain  Gain=1/V_b
  Gain{2..5} (4 alike) : Gain  Gain=I_b
  Gain6 : Gain  Gain=w_b
  Gain7 : Gain  Gain=-1
  Gain8 : Gain  Gain=-1
  Gain9 : Gain  Gain=1/V_b
  Icircd* : Constant  Value=0
  Icircq* : Constant  Value=0
  PID Controller : slpidlib/PID Controller  Controller=PI  Form=Parallel  TimeDomain=Discrete-time  UseExternalTs=off  SampleTime=-1  IntegratorMethod=Forward Euler  FilterMethod=Forward Euler  ControllerParametersSource=internal  P=kpcir  I=kicir  UseKiTs=off  D=0  UseExternalDerivativeSource=off  N=100  UseFilter=on  TunerSelectOption=Transfer Function Based (PID Tuner App)  InitialConditionSource=internal  InitialConditionForIntegrator=0  InitialConditionForFilter=0  DifferentiatorICPrevScaledInput=0  ExternalReset=none  TrackingMode=off  Kt=1  LimitOutput=off  SatLimitsSource=internal  UpperSaturationLimit=inf  LowerSaturationLimit=-inf  LinearizeAsGain=on  AntiWindupMode=none  Kb=1  LimitIntegrator=off  UpperIntegratorSaturationLimit=inf  LowerIntegratorSaturationLimit=-inf  POutMin=[]  POutMax=[]  IOutMin=[]  IOutMax=[]  DOutMin=[]  DOutMax=[]  NOutMin=[]  NOutMax=[]  SumOutMin=[]  SumOutMax=[]  SaturationOutMin=[]  SaturationOutMax=[]  PParamMin=[]  PParamMax=[]  IParamMin=[]  IParamMax=[]  DParamMin=[]  DParamMax=[]  NParamMin=[]  NParamMax=[]  KbParamMin=[]  KbParamMax=[]  KtParamMin=[]  KtParamMax=[]  KbOutMin=[]  KbOutMax=[]  KtOutMin=[]  KtOutMax=[]  IntegratorOutMin=[]  IntegratorOutMax=[]  FilterOutMin=[]  FilterOutMax=[]  SumI1OutMin=[]  SumI1OutMax=[]  SumI2OutMin=[]  SumI2OutMax=[]  SumI3OutMin=[]  SumI3OutMax=[]  SumI4OutMin=[]  SumI4OutMax=[]  SumDOutMin=[]  SumDOutMax=[]  DifferentiatorOutMin=[]  DifferentiatorOutMax=[]  FilterDiffOutCoefMin=[]  FilterDiffOutCoefMax=[]  ReciprocalOutMin=[]  ReciprocalOutMax=[]  SumDenOutMin=[]  SumDenOutMax=[]  SumNumOutMin=[]  SumNumOutMax=[]  DivideOutMin=[]  DivideOutMax=[]  UdiffTsProdOutMin=[]  UdiffTsProdOutMax=[]  NTsProdOutMin=[]  NTsProdOutMax=[]  UintegralTsProdOutMin=[]  UintegralTsProdOutMax=[]  UngainTsProdOutMin=[]  UngainTsProdOutMax=[]  ClampingZeroOutDataTypeStr=Inherit: Inherit via back propagation  ClampingZeroOutMin=[]  ClampingZeroOutMax=[]  FilterDenConstantOutDataTypeStr=Inherit: Inherit via back propagation  FilterDenConstantOutMin=[]  FilterDenConstantOutMax=[]  PCopyOutDataTypeStr=Inherit: Inherit via back propagation  PCopyOutMin=[]  PCopyOutMax=[]  NCopyOutDataTypeStr=Inherit: Inherit via back propagation  NCopyOutMin=[]  NCopyOutMax=[]  IntegratorContinuousStateAttributes=''  IntegratorStateMustResolveToSignalObject=off  IntegratorRTWStateStorageClass=Auto  FilterContinuousStateAttributes=''  FilterStateMustResolveToSignalObject=off  FilterRTWStateStorageClass=Auto  ParallelPVariant=InternalParameters  IdealPVariant=Disabled  IVariant=InternalParameters  DVariant=Disabled  IntegratorVariant=Discrete  SatVariant=Disabled  AWVariant=Passthrough  PCopyVariant=Disabled  TRVariant=Disabled  FdbkBlocksVariant=Forward  IdealPFdbkVariant=Disabled  SatFdbkVariant=Disabled  DerivativeFilterVariant=Disabled  NVariant=Disabled  NCopyVariant=Disabled_SignalSpec  FilterICVariant=Disabled  IntegratorICVariant=InternalICs  ExternalResetVariant=Disabled  TRSumVariant=Passthrough  SumFdbkVariant=Disabled  SumVariant=Sum_PI  TsampFilterVariant=InternalTs  TsampNgainVariant=Passthrough  TsampIntegralVariant=Disabled_SignalSpec  ExternalSaturationOutDataTypeStr=Inherit: Same as second input  DerivativeSourceVariant=Disabled  PreIntVariant=InternalPreInt
  PID Controller1 : slpidlib/PID Controller  Controller=PI  Form=Parallel  TimeDomain=Discrete-time  UseExternalTs=off  SampleTime=-1  IntegratorMethod=Forward Euler  FilterMethod=Forward Euler  ControllerParametersSource=internal  P=kpcir  I=kicir  UseKiTs=off  D=0  UseExternalDerivativeSource=off  N=100  UseFilter=on  TunerSelectOption=Transfer Function Based (PID Tuner App)  InitialConditionSource=internal  InitialConditionForIntegrator=0  InitialConditionForFilter=0  DifferentiatorICPrevScaledInput=0  ExternalReset=none  TrackingMode=off  Kt=1  LimitOutput=off  SatLimitsSource=internal  UpperSaturationLimit=inf  LowerSaturationLimit=-inf  LinearizeAsGain=on  AntiWindupMode=none  Kb=1  LimitIntegrator=off  UpperIntegratorSaturationLimit=inf  LowerIntegratorSaturationLimit=-inf  POutMin=[]  POutMax=[]  IOutMin=[]  IOutMax=[]  DOutMin=[]  DOutMax=[]  NOutMin=[]  NOutMax=[]  SumOutMin=[]  SumOutMax=[]  SaturationOutMin=[]  SaturationOutMax=[]  PParamMin=[]  PParamMax=[]  IParamMin=[]  IParamMax=[]  DParamMin=[]  DParamMax=[]  NParamMin=[]  NParamMax=[]  KbParamMin=[]  KbParamMax=[]  KtParamMin=[]  KtParamMax=[]  KbOutMin=[]  KbOutMax=[]  KtOutMin=[]  KtOutMax=[]  IntegratorOutMin=[]  IntegratorOutMax=[]  FilterOutMin=[]  FilterOutMax=[]  SumI1OutMin=[]  SumI1OutMax=[]  SumI2OutMin=[]  SumI2OutMax=[]  SumI3OutMin=[]  SumI3OutMax=[]  SumI4OutMin=[]  SumI4OutMax=[]  SumDOutMin=[]  SumDOutMax=[]  DifferentiatorOutMin=[]  DifferentiatorOutMax=[]  FilterDiffOutCoefMin=[]  FilterDiffOutCoefMax=[]  ReciprocalOutMin=[]  ReciprocalOutMax=[]  SumDenOutMin=[]  SumDenOutMax=[]  SumNumOutMin=[]  SumNumOutMax=[]  DivideOutMin=[]  DivideOutMax=[]  UdiffTsProdOutMin=[]  UdiffTsProdOutMax=[]  NTsProdOutMin=[]  NTsProdOutMax=[]  UintegralTsProdOutMin=[]  UintegralTsProdOutMax=[]  UngainTsProdOutMin=[]  UngainTsProdOutMax=[]  ClampingZeroOutDataTypeStr=Inherit: Inherit via back propagation  ClampingZeroOutMin=[]  ClampingZeroOutMax=[]  FilterDenConstantOutDataTypeStr=Inherit: Inherit via back propagation  FilterDenConstantOutMin=[]  FilterDenConstantOutMax=[]  PCopyOutDataTypeStr=Inherit: Inherit via back propagation  PCopyOutMin=[]  PCopyOutMax=[]  NCopyOutDataTypeStr=Inherit: Inherit via back propagation  NCopyOutMin=[]  NCopyOutMax=[]  IntegratorContinuousStateAttributes=''  IntegratorStateMustResolveToSignalObject=off  IntegratorRTWStateStorageClass=Auto  FilterContinuousStateAttributes=''  FilterStateMustResolveToSignalObject=off  FilterRTWStateStorageClass=Auto  ParallelPVariant=InternalParameters  IdealPVariant=Disabled  IVariant=InternalParameters  DVariant=Disabled  IntegratorVariant=Discrete  SatVariant=Disabled  AWVariant=Passthrough  PCopyVariant=Disabled  TRVariant=Disabled  FdbkBlocksVariant=Forward  IdealPFdbkVariant=Disabled  SatFdbkVariant=Disabled  DerivativeFilterVariant=Disabled  NVariant=Disabled  NCopyVariant=Disabled_SignalSpec  FilterICVariant=Disabled  IntegratorICVariant=InternalICs  ExternalResetVariant=Disabled  TRSumVariant=Passthrough  SumFdbkVariant=Disabled  SumVariant=Sum_PI  TsampFilterVariant=InternalTs  TsampNgainVariant=Passthrough  TsampIntegralVariant=Disabled_SignalSpec  ExternalSaturationOutDataTypeStr=Inherit: Same as second input  DerivativeSourceVariant=Disabled  PreIntVariant=InternalPreInt
  Product : Product
  Product1 : Product
  Sum : Sum  Inputs=|+-
  Sum1 : Sum  Inputs=|--
  Sum2 : Sum  Inputs=-+|
  Sum3 : Sum  Inputs=+-|
  ucommd* : Outport
  ucommq* : Outport  Port=2
  wires:
  Icircd*/1 -> Sum/1
  Sum/1 -> Gain2/1
  Icircd/1 -> Gain3/1, Sum/2
  Icircq/1 -> Gain4/1, Sum2/1
  Icircq*/1 -> Sum2/2
  Sum2/1 -> Gain5/1
  PID Controller1/1 -> Sum3/2
  PID Controller/1 -> Sum1/1
  w/1 -> Gain6/1
  Product/1 -> Gain/1
  Product1/1 -> Gain1/1
  Sum1/1 -> Gain9/1
  Sum3/1 -> Gain10/1
  Gain/1 -> Sum3/1
  Gain1/1 -> Sum1/2
  Gain2/1 -> PID Controller/1
  Gain3/1 -> Product/1
  Gain6/1 -> Product1/1, Product/2
  Gain4/1 -> Product1/2
  Gain5/1 -> PID Controller1/1
  Gain9/1 -> Gain8/1
  Gain10/1 -> Gain7/1
  Gain8/1 -> ucommd*/1
  Gain7/1 -> ucommq*/1

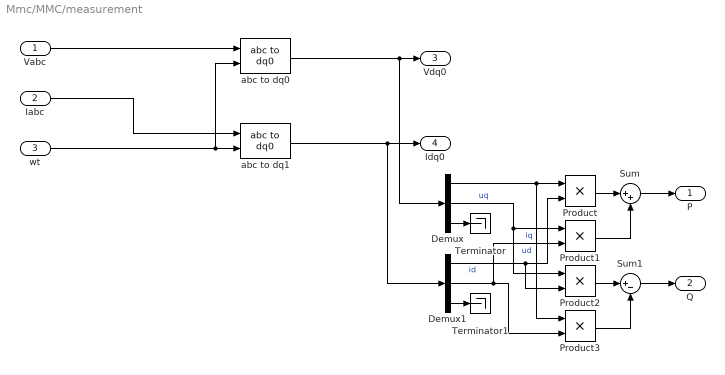
== system Mmc/MMC/measurement ==
  Vabc : Inport
  Iabc : Inport  Port=2
  wt : Inport  Port=3
  Demux : Demux  Outputs=3
  Demux1 : Demux  Outputs=3
  Product{,1..3} (4 alike) : Product
  Sum : Sum  Inputs=|++
  Sum1 : Sum  Inputs=|+-
  Terminator : Terminator
  Terminator1 : Terminator
  abc to dq0 : spsabctodq0Lib/abc to dq0  Alignment=90 degrees behind phase A axis
  abc to dq1 : spsabctodq0Lib/abc to dq0  Alignment=90 degrees behind phase A axis
  P : Outport
  Q : Outport  Port=2
  Vdq0 : Outport  Port=3
  Idq0 : Outport  Port=4
  wires:
  wt/1 -> abc to dq0/2, abc to dq1/2
  Vabc/1 -> abc to dq0/1
  Iabc/1 -> abc to dq1/1
  Demux/3 -> Terminator/1
  Demux1/3 -> Terminator1/1
  Demux/1 -> Product3/1, Product/1  "ud"
  Demux/2 -> Product1/1, Product2/1  "uq"
  Demux1/2 -> Product1/2, Product3/2  "iq"
  Product/1 -> Sum/1
  Product1/1 -> Sum/2
  Product2/1 -> Sum1/1
  Product3/1 -> Sum1/2
  Demux1/1 -> Product2/2, Product/2  "id"
  abc to dq0/1 -> Demux/1, Vdq0/1
  abc to dq1/1 -> Demux1/1, Idq0/1
  Sum/1 -> P/1
  Sum1/1 -> Q/1

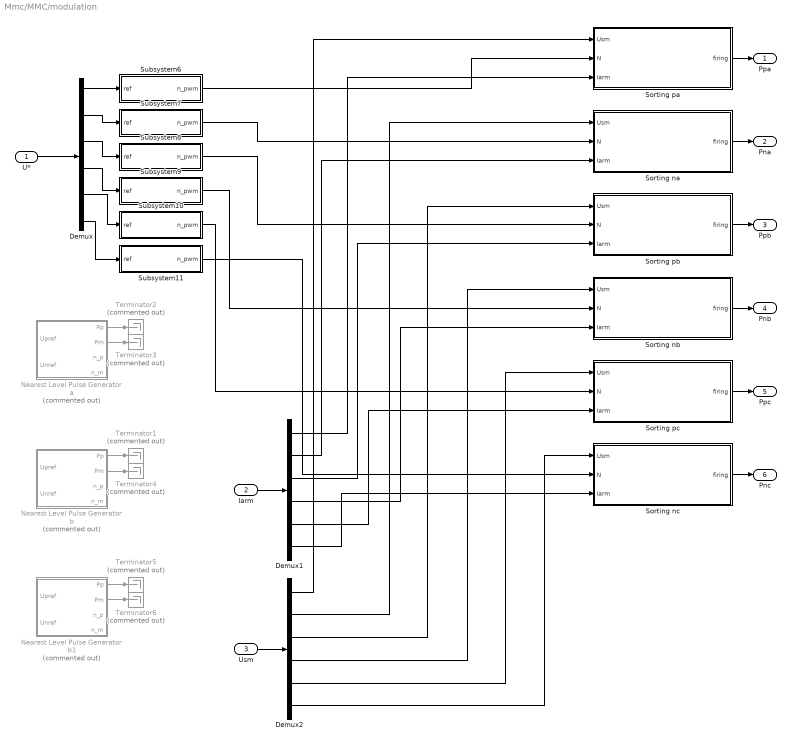
== system Mmc/MMC/modulation ==
  U* : Inport
  Iarm : Inport  Port=2
  Usm : Inport  Port=3
  Demux : Demux  Outputs=6
  Demux1 : Demux  Outputs=6
  Demux2 : Demux  Outputs=6
  "Nearest Level Pulse Generator a " : Subsystem  Commented=on
  Nearest Level Pulse Generator b : Subsystem  Commented=on
  Nearest Level Pulse Generator b1 : Subsystem  Commented=on
  Sorting na : Subsystem
  Sorting nb : Subsystem
  Sorting nc : Subsystem
  Sorting pa : Subsystem
  Sorting pb : Subsystem
  Sorting pc : Subsystem
  Subsystem10 : Subsystem
  Subsystem11 : Subsystem
  Subsystem6 : Subsystem
  Subsystem7 : Subsystem
  Subsystem8 : Subsystem
  Subsystem9 : Subsystem
  Terminator{1..6} (6 alike) : Terminator  Commented=on
  Ppa : Outport
  Pna : Outport  Port=2
  Ppb : Outport  Port=3
  Pnb : Outport  Port=4
  Ppc : Outport  Port=5
  Pnc : Outport  Port=6
  wires:
  Sorting pa/1(firing) -> Ppa/1
  Sorting na/1(firing) -> Pna/1
  Sorting pb/1(firing) -> Ppb/1
  Sorting nb/1(firing) -> Pnb/1
  Sorting nc/1(firing) -> Pnc/1
  Sorting pc/1(firing) -> Ppc/1
  Iarm/1 -> Demux1/1
  Demux1/1 -> Sorting pa/3(Iarm)
  Demux1/2 -> Sorting na/3(Iarm)
  Demux1/3 -> Sorting pb/3(Iarm)
  Demux1/4 -> Sorting nb/3(Iarm)
  Demux1/5 -> Sorting pc/3(Iarm)
  Demux1/6 -> Sorting nc/3(Iarm)
  Usm/1 -> Demux2/1
  Demux2/6 -> Sorting nc/1(Usm)
  Demux2/5 -> Sorting pc/1(Usm)
  Demux2/4 -> Sorting nb/1(Usm)
  Demux2/3 -> Sorting pb/1(Usm)
  Demux2/2 -> Sorting na/1(Usm)
  Demux2/1 -> Sorting pa/1(Usm)
  U*/1 -> Demux/1
  Demux/1 -> Subsystem6/1(ref)
  Demux/5 -> Subsystem10/1(ref)
  Demux/6 -> Subsystem11/1(ref)
  Demux/3 -> Subsystem8/1(ref)
  Demux/4 -> Subsystem9/1(ref)
  Demux/2 -> Subsystem7/1(ref)
  Nearest Level Pulse Generator b1/2(Pm) -> Terminator6/1
  "Nearest Level Pulse Generator a "/1(Pp) -> Terminator2/1
  Nearest Level Pulse Generator b/2(Pm) -> Terminator4/1
  Nearest Level Pulse Generator b1/1(Pp) -> Terminator5/1
  "Nearest Level Pulse Generator a "/2(Pm) -> Terminator3/1
  Nearest Level Pulse Generator b/1(Pp) -> Terminator1/1
  Subsystem6/1(n_pwm) -> Sorting pa/2(N)
  Subsystem7/1(n_pwm) -> Sorting na/2(N)
  Subsystem8/1(n_pwm) -> Sorting pb/2(N)
  Subsystem9/1(n_pwm) -> Sorting nb/2(N)
  Subsystem10/1(n_pwm) -> Sorting pc/2(N)
  Subsystem11/1(n_pwm) -> Sorting nc/2(N)

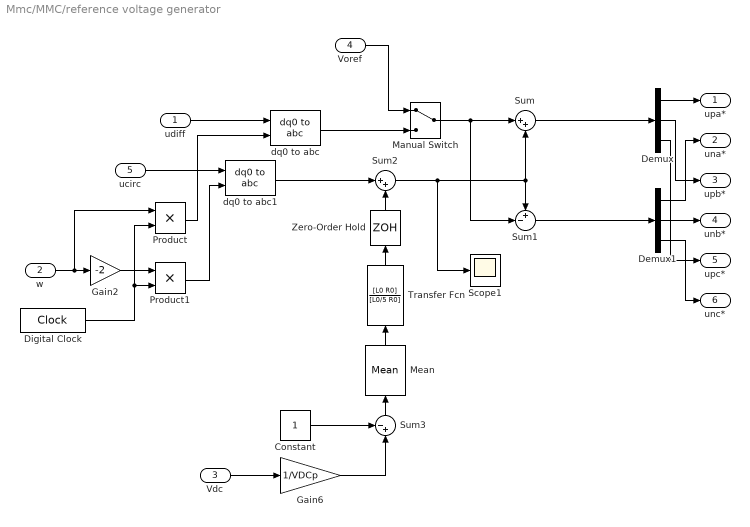
== system Mmc/MMC/reference voltage generator ==
  udiff : Inport
  w : Inport  Port=2
  Vdc : Inport  Port=3
  Voref : Inport  Port=4
  ucirc : Inport  Port=5
  Constant : Constant
  Demux : Demux  Outputs=3
  Demux1 : Demux  Outputs=3
  Digital Clock : DigitalClock  SampleTime=Ts_Power
  Gain2 : Gain  Gain=-2
  Gain6 : Gain  Gain=1/VDCp
  Manual Switch : ManualSwitch
  Mean : spsMeanLib/Mean  Freq=Fnom  Vinit=0  Ts=Ts_Power
  Product : Product
  Product1 : Product
  Scope1 : Scope
  Sum : Sum  Inputs=|++
  Sum1 : Sum  Inputs=+-|
  Sum2 : Sum  Inputs=|++
  Sum3 : Sum  Inputs=-+|
  Transfer Fcn : TransferFcn  Numerator=[L0 R0]  Denominator=[L0/5 R0]
  Zero-Order Hold : ZeroOrderHold  SampleTime=Ts_Power
  dq0 to abc : spsdq0toabcLib/dq0 to abc  Alignment=90 degrees behind phase A axis
  dq0 to abc1 : spsdq0toabcLib/dq0 to abc  Alignment=90 degrees behind phase A axis
  upa* : Outport
  una* : Outport  Port=2
  upb* : Outport  Port=3
  unb* : Outport  Port=4
  upc* : Outport  Port=5
  unc* : Outport  Port=6
  wires:
  Demux/1 -> upa*/1
  Demux/2 -> upb*/1
  Demux/3 -> upc*/1
  Demux1/1 -> una*/1
  Demux1/2 -> unb*/1
  Demux1/3 -> unc*/1
  w/1 -> Product/1, Gain2/1
  Gain2/1 -> Product1/1
  Transfer Fcn/1 -> Zero-Order Hold/1
  Constant/1 -> Sum3/1
  Sum2/1 -> Scope1/1, Sum/2, Sum1/1
  Product1/1 -> dq0 to abc1/2
  Sum3/1 -> Mean/1
  Vdc/1 -> Gain6/1
  Digital Clock/1 -> Product/2, Product1/2
  Product/1 -> dq0 to abc/2
  Gain6/1 -> Sum3/2
  Mean/1 -> Transfer Fcn/1
  Sum1/1 -> Demux1/1
  Sum/1 -> Demux/1
  Manual Switch/1 -> Sum1/2, Sum/1
  Voref/1 -> Manual Switch/1
  Zero-Order Hold/1 -> Sum2/2
  dq0 to abc/1 -> Manual Switch/2
  ucirc/1 -> dq0 to abc1/1
  udiff/1 -> dq0 to abc/1
  dq0 to abc1/1 -> Sum2/1

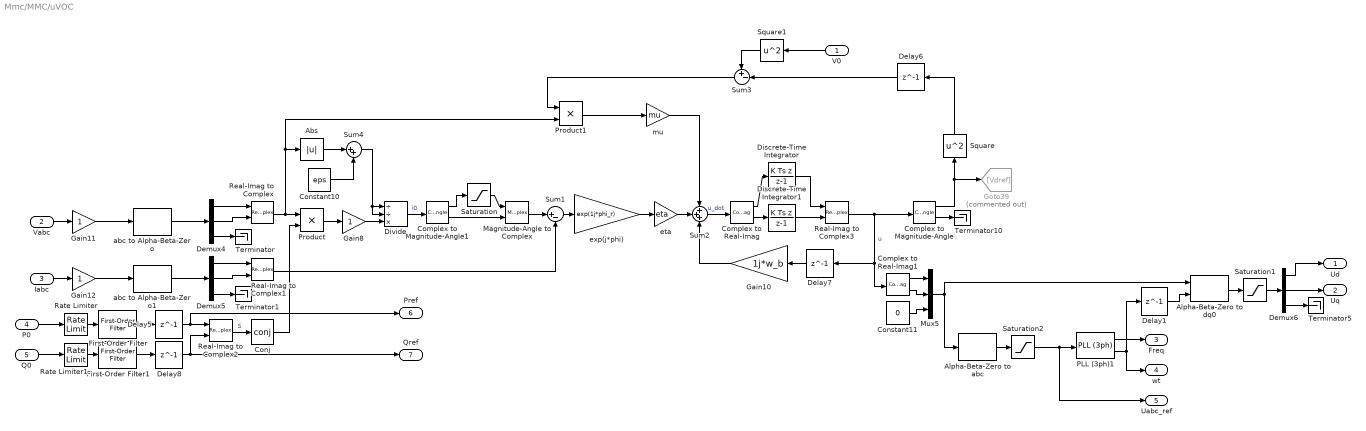
== system Mmc/MMC/uVOC ==
  V0 : Inport
  Vabc : Inport  Port=2
  Iabc : Inport  Port=3
  P0 : Inport  Port=4
  Q0 : Inport  Port=5
  Abs : Abs  SaturateOnIntegerOverflow=off
  Alpha-Beta-Zero to abc : spsAlphaBetaZerotoabcLib/Alpha-Beta-Zero to abc
      settings: LibrarySourceBlock=|
      | sps_lib/Control/Alpha-Beta-Zero
      | to abc
  Alpha-Beta-Zero to dq0 : spsAlphaBetaZerotodq0Lib/Alpha-Beta-Zero to dq0  Alignment=90 degrees behind phase A axis
  Complex to Magnitude-Angle : ComplexToMagnitudeAngle
  Complex to Magnitude-Angle1 : ComplexToMagnitudeAngle
  Complex to Real-Imag : ComplexToRealImag
  Complex to Real-Imag1 : ComplexToRealImag
  Conj : Math  Operator=conj
  Constant10 : Constant  Value=eps  SampleTime=Ts_Power
  Constant11 : Constant  Value=0  SampleTime=Ts_Power
  Delay1 : Delay  DelayLength=1  InitialCondition=50  InputProcessing=Columns as channels (frame based)  SampleTime=Ts_Power
  Delay5 : Delay  DelayLength=1  InputProcessing=Columns as channels (frame based)  SampleTime=Ts_Power
  Delay6 : Delay  DelayLength=1  InitialCondition=1  InputProcessing=Columns as channels (frame based)
  Delay7 : Delay  DelayLength=1  InputProcessing=Columns as channels (frame based)
  Delay8 : Delay  DelayLength=1  InputProcessing=Columns as channels (frame based)  SampleTime=Ts_Power
  Demux4 : Demux  Outputs=3
  Demux5 : Demux  Outputs=3
  Demux6 : Demux  Outputs=3
  Discrete-Time Integrator : DiscreteIntegrator  IntegratorMethod=Integration: Backward Euler  SampleTime=-1  ICPrevOutput=DiscIntNeverNeededParam  ICPrevScaledInput=DiscIntNeverNeededParam
  Discrete-Time Integrator1 : DiscreteIntegrator  IntegratorMethod=Integration: Backward Euler  InitialCondition=-1  SampleTime=-1  ICPrevOutput=DiscIntNeverNeededParam  ICPrevScaledInput=DiscIntNeverNeededParam
  Divide : Product  Inputs=//*
  First-Order Filter : spsFirstOrderFilterLib/First-Order Filter  FilterType=Lowpass  Tc=1.5/Fnom  Ts=Ts_Power  Initialize=on  Vac_Init=[0, 0, 0]  Vdc_Init=0  PlotResponse=off  FreqRange="[0,  200,  1]"
  First-Order Filter1 : spsFirstOrderFilterLib/First-Order Filter  FilterType=Lowpass  Tc=1.5/Fnom  Ts=Ts_Power  Initialize=on  Vac_Init=[0, 0, 0]  Vdc_Init=0  PlotResponse=off  FreqRange="[0,  200,  1]"
  Gain10 : Gain  Gain=1j*w_b
  Gain11 : Gain
  Gain12 : Gain
  Gain8 : Gain
  Goto39 : Goto  Commented=on  GotoTag=Vdref
  Magnitude-Angle to Complex : MagnitudeAngleToComplex
  Mux5 : Mux  Inputs=3
  PLL (3ph)1 : spsPLL3phLib/PLL (3ph)  Fmin=45  Par_Init=[0, 50]  ParK=[9.2/.18 (4.6/.18/.8)^2 0]  TcD=1e-4  MaxRateChangeFreq=20  FilterCutOffFreq=80  Ts=Ts_Power  AGC=on
  Product : Product
  Product1 : Product
  Rate Limiter : RateLimiter  RisingSlewLimit=10  FallingSlewLimit=-10  SampleTimeMode=inherited
  Rate Limiter1 : RateLimiter  RisingSlewLimit=10  FallingSlewLimit=-10  SampleTimeMode=inherited
  Real-Imag to Complex{,1..3} (4 alike) : RealImagToComplex
  Saturation : Saturate  UpperLimit=1.2  LowerLimit=-1.2
  Saturation1 : Saturate  UpperLimit=2  LowerLimit=-2
  Saturation2 : Saturate  UpperLimit=2  LowerLimit=-2
  Square : Math  Operator=square
  Square1 : Math  Operator=square
  Sum1 : Sum  Inputs=|+-
  Sum2 : Sum  Inputs=+++
  Sum3 : Sum  Inputs=+-|
  Sum4 : Sum  Inputs=|++
  Terminator{,1,5,10} (4 alike) : Terminator
  abc to Alpha-Beta-Zero : spsabctoAlphaBetaZeroLib/abc to Alpha-Beta-Zero
  abc to Alpha-Beta-Zero1 : spsabctoAlphaBetaZeroLib/abc to Alpha-Beta-Zero
  eta : Gain  Gain=eta
  exp(j*phi) : Gain  Gain=exp(1j*phi_r)
  mu : Gain  Gain=mu
  Ud : Outport
  Uq : Outport  Port=2
  Freq : Outport  Port=3
  wt : Outport  Port=4
  Uabc_ref : Outport  Port=5
  Pref : Outport  Port=6
  Qref : Outport  Port=7
  wires:
  Real-Imag to Complex/1 -> Product1/2, Abs/1, Product/1
  Constant11/1 -> Mux5/3
  Alpha-Beta-Zero to dq0/1 -> Saturation1/1
  abc to Alpha-Beta-Zero1/1 -> Demux5/1
  Delay7/1 -> Gain10/1
  exp(j*phi)/1 -> eta/1
  Real-Imag to Complex3/1 -> Complex to Real-Imag1/1, Delay7/1, Complex to Magnitude-Angle/1  "u"
  Conj/1 -> Product/2
  First-Order Filter/1 -> Delay5/1
  Delay6/1 -> Sum3/2
  Abs/1 -> Sum4/1
  Demux6/1 -> Ud/1
  Iabc/1 -> Gain12/1
  Square1/1 -> Sum3/1
  Demux5/2 -> Real-Imag to Complex1/2
  Demux5/3 -> Terminator1/1
  abc to Alpha-Beta-Zero/1 -> Demux4/1
  Product/1 -> Gain8/1
  First-Order Filter1/1 -> Delay8/1
  Real-Imag to Complex1/1 -> Sum1/2
  Complex to Real-Imag/2 -> Discrete-Time Integrator1/1
  Demux4/3 -> Terminator/1
  Complex to Magnitude-Angle/1 -> Goto39/1, Square/1
  Gain8/1 -> Divide/3
  Delay8/1 -> Real-Imag to Complex2/2, Qref/1
  Demux5/1 -> Real-Imag to Complex1/1
  Gain12/1 -> abc to Alpha-Beta-Zero1/1
  Complex to Magnitude-Angle/2 -> Terminator10/1
  Complex to Real-Imag1/1 -> Mux5/1
  Demux4/1 -> Real-Imag to Complex/1
  V0/1 -> Square1/1
  Complex to Real-Imag/1 -> Discrete-Time Integrator/1
  PLL (3ph)1/2 -> wt/1, Delay1/1
  Sum2/1 -> Complex to Real-Imag/1  "u_dot"
  eta/1 -> Sum2/2
  Gain11/1 -> abc to Alpha-Beta-Zero/1
  Product1/1 -> mu/1
  Sum1/1 -> exp(j*phi)/1
  Sum3/1 -> Product1/1
  Gain10/1 -> Sum2/3
  Delay5/1 -> Pref/1, Real-Imag to Complex2/1
  Alpha-Beta-Zero to abc/1 -> Saturation2/1
  Complex to Real-Imag1/2 -> Mux5/2
  Demux4/2 -> Real-Imag to Complex/2
  Demux6/3 -> Terminator5/1
  Real-Imag to Complex2/1 -> Conj/1  "S"
  Vabc/1 -> Gain11/1
  Demux6/2 -> Uq/1
  PLL (3ph)1/1 -> Freq/1
  Discrete-Time Integrator/1 -> Real-Imag to Complex3/1
  Discrete-Time Integrator1/1 -> Real-Imag to Complex3/2
  Square/1 -> Delay6/1
  Mux5/1 -> Alpha-Beta-Zero to dq0/1, Alpha-Beta-Zero to abc/1
  Saturation2/1 -> Uabc_ref/1, PLL (3ph)1/1
  Saturation1/1 -> Demux6/1
  Delay1/1 -> Alpha-Beta-Zero to dq0/2
  Rate Limiter/1 -> First-Order Filter/1
  Rate Limiter1/1 -> First-Order Filter1/1
  Complex to Magnitude-Angle1/1 -> Saturation/1
  Saturation/1 -> Magnitude-Angle to Complex/1
  Complex to Magnitude-Angle1/2 -> Magnitude-Angle to Complex/2
  Constant10/1 -> Sum4/2
  Sum4/1 -> Divide/2, Divide/1
  P0/1 -> Rate Limiter/1
  Q0/1 -> Rate Limiter1/1
  Divide/1 -> Complex to Magnitude-Angle1/1  "i0"
  Magnitude-Angle to Complex/1 -> Sum1/1
  mu/1 -> Sum2/1

== system Mmc/MMC/Full-bridge/HBua1 ==
  gates : Inport
  Ch : spsSeriesRLCBranchLib/Series RLC Branch  LConnTagsString=__new0  RConnTagsString=__new0  BranchType=RC  Resistance=Rh(2,1)  Inductance=1e-3  SetiL0=off  InitialCurrent=0  Capacitance=Ch(2,1)  Setx0=off  InitialVoltage=750  Measurements=None
  Cm : spsSeriesRLCBranchLib/Series RLC Branch  LConnTagsString=__new0  RConnTagsString=__new0  BranchType=RC  Resistance=Rm(2,1)  Inductance=1e-3  SetiL0=off  InitialCurrent=0  Capacitance=Cmo(2,1)  Setx0=on  InitialVoltage=20  Measurements=None
  Demux1 : Demux
  IGBT/Diode{,1..3} (4 alike) : spsIGBTDiodeLib/IGBT//Diode  Ron=Ron  Rs=Rs  Cs=Cs  Measurements=off
  Rdis : spsSeriesRLCBranchLib/Series RLC Branch  LConnTagsString=__new0  RConnTagsString=__new0  BranchType=R  Resistance=Rdis(2,1)  Inductance=1e-3  SetiL0=off  InitialCurrent=0  Capacitance=Cm  Setx0=off  InitialVoltage=750  Measurements=None
  VA : PMIOPort  Side=Left
  VB : PMIOPort  Port=2  Side=Left
  DC+ : PMIOPort  Port=3  Side=Right
  DC- : PMIOPort  Port=4  Side=Right
  wires:
  gates/1 -> Demux1/1
  Demux1/4 -> IGBT/Diode3/1
  Demux1/3 -> IGBT/Diode2/1
  Demux1/2 -> IGBT/Diode1/1
  Demux1/1 -> IGBT/Diode/1
  connections:
  IGBT/Diode3/LConn1 -- VB/RConn1 -- IGBT/Diode2/RConn1
  Ch/LConn1 -- Rdis/LConn1 -- DC+/RConn1 -- IGBT/Diode/LConn1 -- IGBT/Diode2/LConn1 -- Cm/LConn1
  IGBT/Diode/RConn1 -- VA/RConn1 -- IGBT/Diode1/LConn1
  Ch/RConn1 -- DC-/RConn1 -- Rdis/RConn1 -- Cm/RConn1 -- IGBT/Diode3/RConn1 -- IGBT/Diode1/RConn1
